simulink model "kuka_IMPC_lev2"  (R2022b)
settings: Solver=ode1  StartTime=0.0  StopTime=T_run  FixedStep=Ts  MaxStep=0.001  MinStep=0.0001  RelTol=1e-3
InitFcn:
  | kuka_IMPC_PriController_simulink_initial
StopFcn:
  | %Analyze%
values from neighbouring files (symbols this model uses):
  Xprime_r_lev1 = [Xprime_r_ini_stop_lev1 Xprime_r_lev1]    [Get_X_ref.m]
undefined symbols (not defined in the file or in its folder): A1_X_bar_lev1, A_QP, B1_dtau_bar_lev1, K_lev1, L1_tilde, L2_tilde, L_lev1, lb_QP, lbA_QP_ini, N, q_bar_sim_ini, q_ini, qd_ini, R_const_lev1, tau_sim_ini, Ts, ub_QP, ubA_QP_ini, x1_bar_sim_ini
libraries: robotmaniplib x8, cjt_library_models x1
settings Model: PauseTimes=7.5  Creator=ywang  LastModifiedBy=zheng
settings SolverCC: InitialStep=0.0001  AlgebraicLoopSolver=LineSearch
settings DataIOCC: ReturnWorkspaceOutputs=off
settings DebuggingCC: UnconnectedInputMsg=warning  UnconnectedOutputMsg=warning  UnconnectedLineMsg=warning  PregeneratedLibrarySubsystemCodeDiagnostic=none  SFMachineParentedDataDiag=warning  ArithmeticOperatorsInVariantConditions=warning
settings ModelReferenceCC: EnableRefExpFcnMdlSchedulingChecks=on
settings SFSimCC: SimUseLocalCustomCode=off  CustomCodeUndefinedFunction=UseInterfaceOnly
settings RTWCC: RTWUseLocalCustomCode=off  DLArmComputeVersion=19.05
settings CodeAppCC: StateflowObjectComments=on

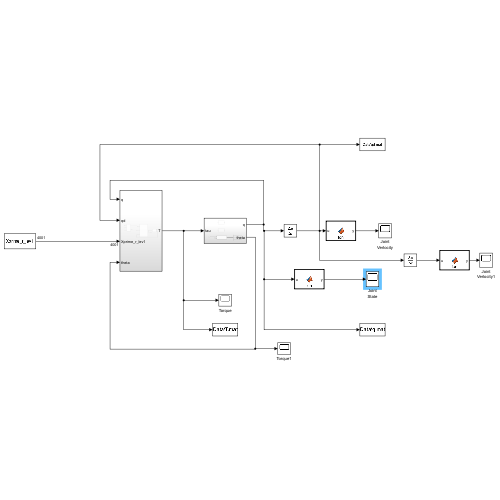
[thumbnail: Simulink's stored preview of the top-level diagram]
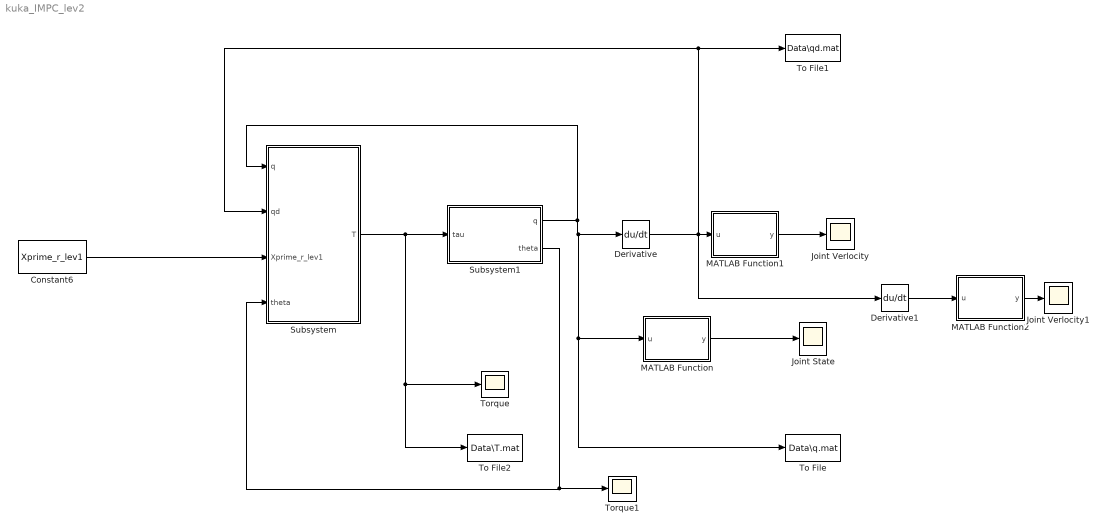
== system kuka_IMPC_lev2 ==
  Constant6 : Constant  Value=Xprime_r_lev1
  Derivative : Derivative
  Derivative1 : Derivative
  Joint State : Scope
  Joint Verlocity : Scope
  Joint Verlocity1 : Scope
  MATLAB Function : MATLAB Function  TreatAsAtomicUnit=on
  MATLAB Function1 : MATLAB Function  TreatAsAtomicUnit=on
  MATLAB Function2 : MATLAB Function  TreatAsAtomicUnit=on
  Subsystem : Subsystem
  Subsystem1 : Subsystem
  To File : ToFile  Filename=Data\q.mat  MatrixName=q
  To File1 : ToFile  Filename=Data\qd.mat  MatrixName=qd
  To File2 : ToFile  Filename=Data\T.mat  MatrixName=T
  Torque : Scope
  Torque1 : Scope
  wires:
  Subsystem/1(T) -> Torque/1, To File2/1, Subsystem1/1(tau)
  Constant6/1 -> Subsystem/3(Xprime_r_lev1)
  Subsystem1/1(q) -> Derivative/1, MATLAB Function/1(u), To File/1, Subsystem/1(q)
  MATLAB Function/1(y) -> Joint State/1
  MATLAB Function1/1(y) -> Joint Verlocity/1
  MATLAB Function2/1(y) -> Joint Verlocity1/1
  Derivative/1 -> Derivative1/1, MATLAB Function1/1(u), To File1/1, Subsystem/2(qd)
  Derivative1/1 -> MATLAB Function2/1(u)
  Subsystem1/2(theta) -> Torque1/1, Subsystem/4(theta)

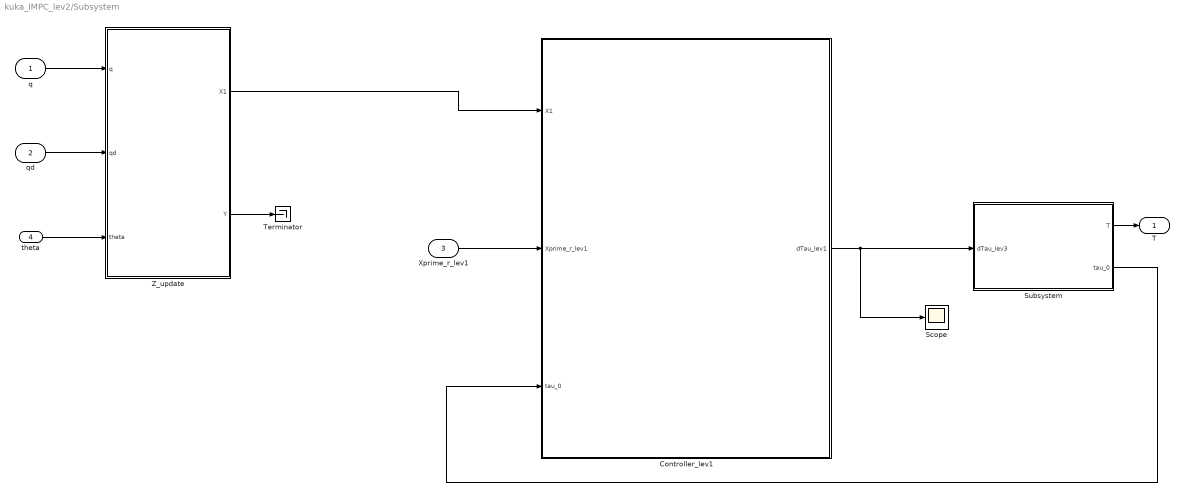
== system kuka_IMPC_lev2/Subsystem ==
  q : Inport
  qd : Inport  Port=2
  Xprime_r_lev1 : Inport  Port=3
  theta : Inport  Port=4
  Controller_lev1 : Subsystem
  Scope : Scope
  Subsystem : Subsystem
  Terminator : Terminator
  Z_update : Subsystem
  T : Outport
  wires:
  q/1 -> Z_update/1(q)
  qd/1 -> Z_update/2(qd)
  Z_update/1(X1) -> Controller_lev1/1(X1)
  Xprime_r_lev1/1 -> Controller_lev1/2(Xprime_r_lev1)
  Subsystem/1(T) -> T/1
  Subsystem/2(tau_0) -> Controller_lev1/3(tau_0)
  Z_update/2(Y) -> Terminator/1
  Controller_lev1/1(dTau_lev1) -> Subsystem/1(dTau_lev3), Scope/1
  theta/1 -> Z_update/3(theta)

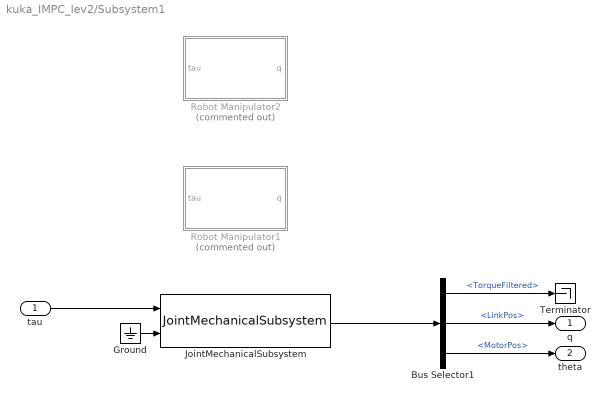
== system kuka_IMPC_lev2/Subsystem1 ==
  tau : Inport
  Bus Selector1 : BusSelector  OutputSignals=TorqueFiltered,LinkPos,MotorPos
  Ground : Ground
  JointMechanicalSubsystem : cjt_library_models/Joint models/JointMechanicalSubsystem  jointObj=exJoint  fc_vel=1000  fc_torque=1000  input_delay=0  output_delay=1  quantize=off  quantize_bits=19  input_noise_enabled=off  output_noise_enabled=off  var_u=0  var_y=1.8e-10
  Robot Manipulator1 : Subsystem  Commented=on
  Robot Manipulator2 : Subsystem  Commented=on
  Terminator : Terminator
  q : Outport
  theta : Outport  Port=2
  wires:
  Bus Selector1/1 -> Terminator/1  "<TorqueFiltered>"
  JointMechanicalSubsystem/1 -> Bus Selector1/1
  Ground/1 -> JointMechanicalSubsystem/2
  tau/1 -> JointMechanicalSubsystem/1
  Bus Selector1/2 -> q/1  "<LinkPos>"
  Bus Selector1/3 -> theta/1  "<MotorPos>"

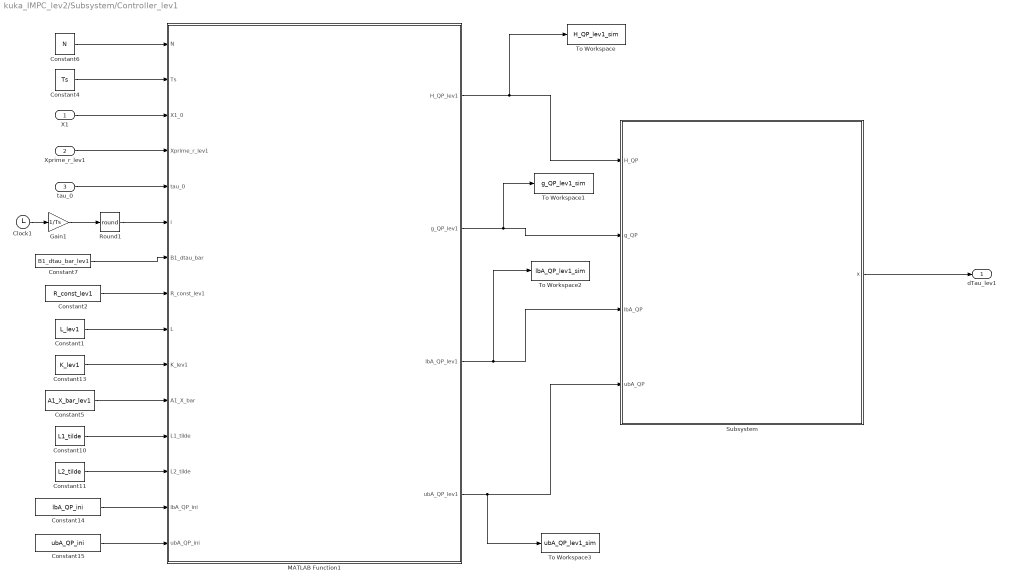
== system kuka_IMPC_lev2/Subsystem/Controller_lev1 ==
  X1 : Inport
  Xprime_r_lev1 : Inport  Port=2
  tau_0 : Inport  Port=3
  Clock1 : Clock
  Constant1 : Constant  Value=L_lev1
  Constant10 : Constant  Value=L1_tilde
  Constant11 : Constant  Value=L2_tilde
  Constant13 : Constant  Value=K_lev1
  Constant14 : Constant  Value=lbA_QP_ini
  Constant15 : Constant  Value=ubA_QP_ini
  Constant2 : Constant  Value=R_const_lev1
  Constant4 : Constant  Value=Ts
  Constant5 : Constant  Value=A1_X_bar_lev1
  Constant6 : Constant  Value=N
  Constant7 : Constant  Value=B1_dtau_bar_lev1
  Gain1 : Gain  Gain=1/Ts
  MATLAB Function1 : MATLAB Function  TreatAsAtomicUnit=on
  Round1 : Rounding  Operator=round
  Subsystem : Subsystem
  To Workspace : ToWorkspace  VariableName=H_QP_lev1_sim  SaveFormat=Timeseries  SampleTime=-1
  To Workspace1 : ToWorkspace  VariableName=g_QP_lev1_sim  SaveFormat=Timeseries  SampleTime=-1
  To Workspace2 : ToWorkspace  VariableName=lbA_QP_lev1_sim  SaveFormat=Timeseries  SampleTime=-1
  To Workspace3 : ToWorkspace  VariableName=ubA_QP_lev1_sim  SaveFormat=Timeseries  SampleTime=-1
  dTau_lev1 : Outport
  wires:
  Constant4/1 -> MATLAB Function1/2(Ts)
  Constant1/1 -> MATLAB Function1/9(L)
  Constant5/1 -> MATLAB Function1/11(A1_X_bar)
  Constant11/1 -> MATLAB Function1/13(L2_tilde)
  Constant10/1 -> MATLAB Function1/12(L1_tilde)
  MATLAB Function1/1(H_QP_lev1) -> To Workspace/1, Subsystem/1(H_QP)
  MATLAB Function1/2(g_QP_lev1) -> To Workspace1/1, Subsystem/2(g_QP)
  Clock1/1 -> Gain1/1
  Gain1/1 -> Round1/1
  Xprime_r_lev1/1 -> MATLAB Function1/4(Xprime_r_lev1)
  Constant13/1 -> MATLAB Function1/10(K_lev1)
  Constant14/1 -> MATLAB Function1/14(lbA_QP_ini)
  Constant15/1 -> MATLAB Function1/15(ubA_QP_ini)
  X1/1 -> MATLAB Function1/3(X1_0)
  tau_0/1 -> MATLAB Function1/5(tau_0)
  Constant6/1 -> MATLAB Function1/1(N)
  Subsystem/1(x) -> dTau_lev1/1
  MATLAB Function1/3(lbA_QP_lev1) -> To Workspace2/1, Subsystem/3(lbA_QP)
  MATLAB Function1/4(ubA_QP_lev1) -> To Workspace3/1, Subsystem/4(ubA_QP)
  Constant7/1 -> MATLAB Function1/7(B1_dtau_bar)
  Constant2/1 -> MATLAB Function1/8(R_const_lev1)
  Round1/1 -> MATLAB Function1/6(i)

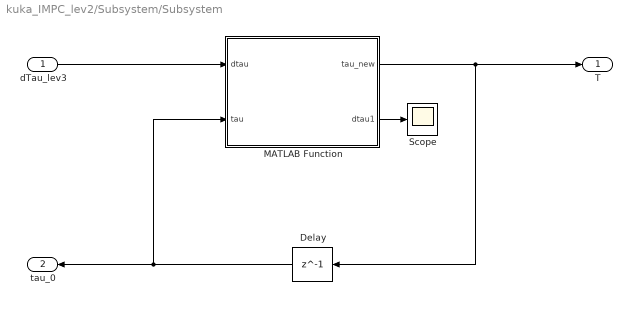
== system kuka_IMPC_lev2/Subsystem/Subsystem ==
  dTau_lev3 : Inport
  Delay : Delay  DelayLength=1  InitialCondition=tau_sim_ini
  MATLAB Function : MATLAB Function  TreatAsAtomicUnit=on
  Scope : Scope
  T : Outport
  tau_0 : Outport  Port=2
  wires:
  dTau_lev3/1 -> MATLAB Function/1(dtau)
  Delay/1 -> tau_0/1, MATLAB Function/2(tau)
  MATLAB Function/1(tau_new) -> Delay/1, T/1
  MATLAB Function/2(dtau1) -> Scope/1

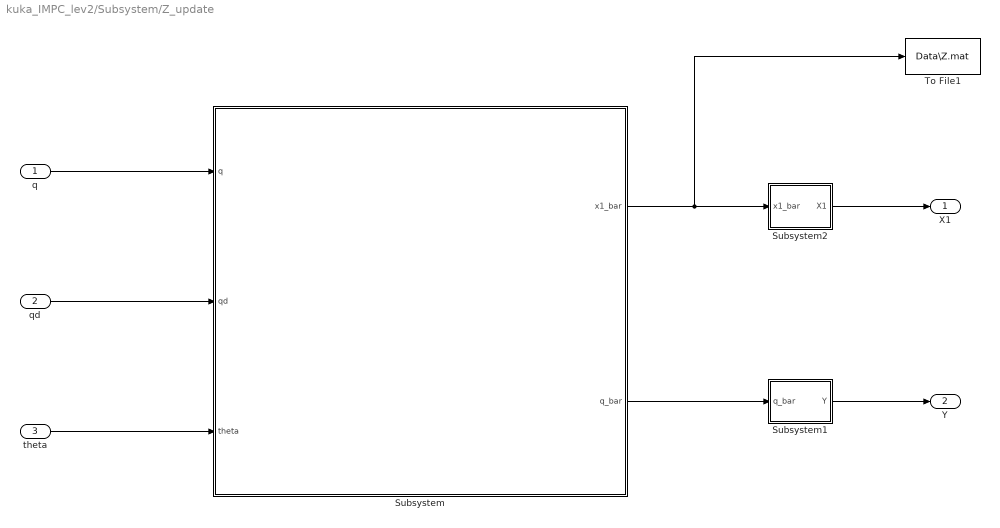
== system kuka_IMPC_lev2/Subsystem/Z_update ==
  q : Inport
  qd : Inport  Port=2
  theta : Inport  Port=3
  Subsystem : Subsystem
  Subsystem1 : Subsystem
  Subsystem2 : Subsystem
  To File1 : ToFile  Filename=Data\Z.mat  MatrixName=Z
  X1 : Outport
  Y : Outport  Port=2
  wires:
  qd/1 -> Subsystem/2(qd)
  q/1 -> Subsystem/1(q)
  Subsystem1/1(Y) -> Y/1
  Subsystem/2(q_bar) -> Subsystem1/1(q_bar)
  Subsystem2/1(X1) -> X1/1
  Subsystem/1(x1_bar) -> To File1/1, Subsystem2/1(x1_bar)
  theta/1 -> Subsystem/3(theta)

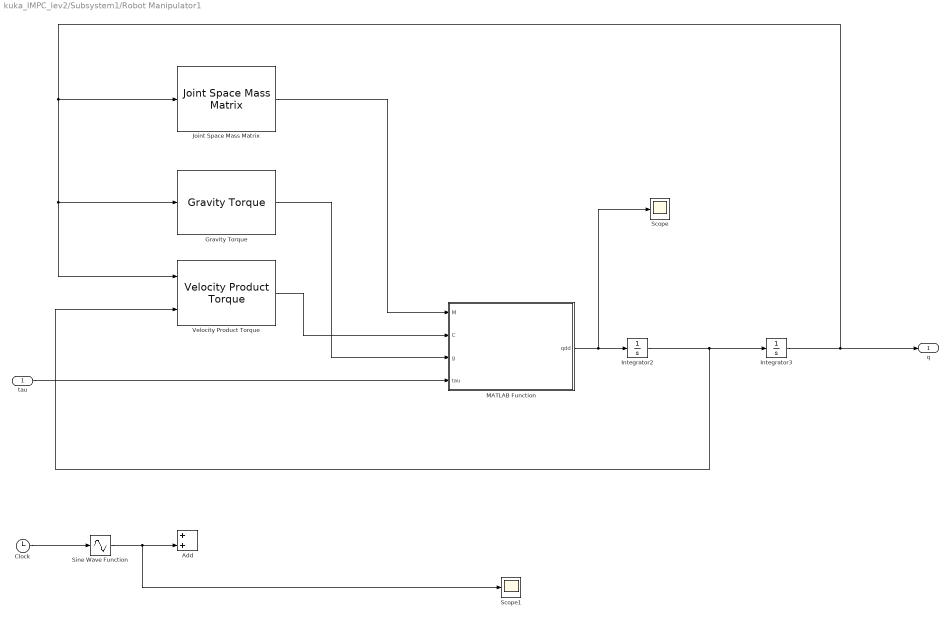
== system kuka_IMPC_lev2/Subsystem1/Robot Manipulator1 ==
  tau : Inport
  Add : Sum
  Clock : Clock
  Gravity Torque : robotmaniplib/Gravity Torque  RigidBodyTree=kuka  SimulateUsing=Interpreted execution
  Integrator2 : Integrator  InitialCondition=qd_ini  ContinuousStateAttributes='velocity'
  Integrator3 : Integrator  InitialCondition=q_ini  ContinuousStateAttributes='position'
  Joint Space Mass Matrix : robotmaniplib/Joint Space Mass Matrix  RigidBodyTree=kuka  SimulateUsing=Interpreted execution
  MATLAB Function : MATLAB Function  TreatAsAtomicUnit=on
  Scope : Scope
  Scope1 : Scope
  Sine Wave Function : Sin  TimeSource=Use external signal  Amplitude=0.5  Frequency=2  SampleTime=0
  Velocity Product Torque : robotmaniplib/Velocity Product Torque  RigidBodyTree=kuka  SimulateUsing=Interpreted execution
  q : Outport  VectorParamsAs1DForOutWhenUnconnected=off
  wires:
  Integrator3/1 -> q/1, Velocity Product Torque/1, Gravity Torque/1, Joint Space Mass Matrix/1
  Integrator2/1 -> Integrator3/1, Velocity Product Torque/2
  Joint Space Mass Matrix/1 -> MATLAB Function/1(M)
  MATLAB Function/1(qdd) -> Scope/1, Integrator2/1
  Velocity Product Torque/1 -> MATLAB Function/2(C)
  Gravity Torque/1 -> MATLAB Function/3(g)
  Sine Wave Function/1 -> Scope1/1, Add/2
  Clock/1 -> Sine Wave Function/1
  tau/1 -> MATLAB Function/4(tau)

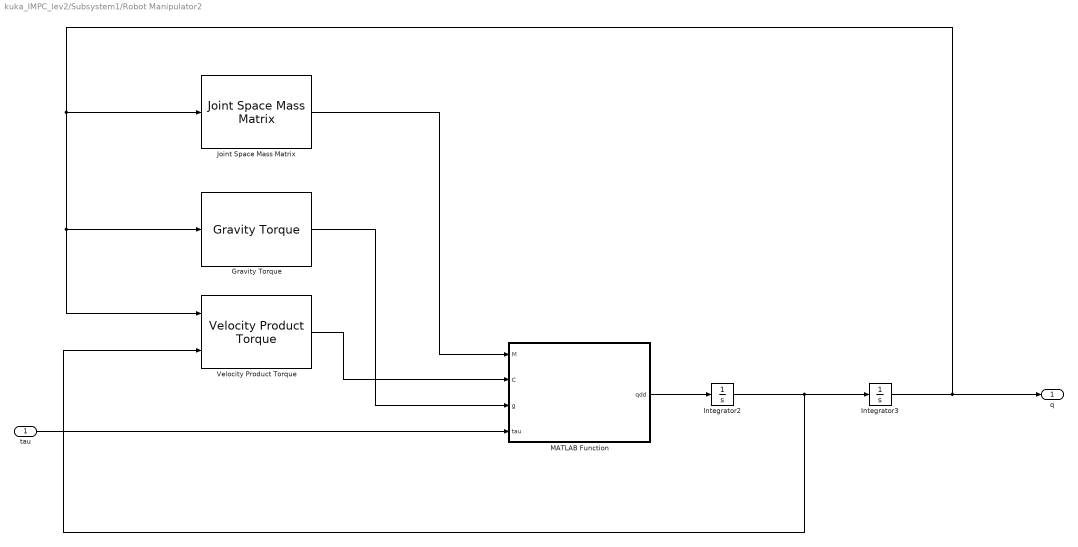
== system kuka_IMPC_lev2/Subsystem1/Robot Manipulator2 ==
  tau : Inport
  Gravity Torque : robotmaniplib/Gravity Torque  RigidBodyTree=kuka  SimulateUsing=Interpreted execution
  Integrator2 : Integrator  InitialCondition=qd_ini  ContinuousStateAttributes='velocity'
  Integrator3 : Integrator  InitialCondition=q_ini  ContinuousStateAttributes='position'
  Joint Space Mass Matrix : robotmaniplib/Joint Space Mass Matrix  RigidBodyTree=kuka  SimulateUsing=Interpreted execution
  MATLAB Function : MATLAB Function  TreatAsAtomicUnit=on
  Velocity Product Torque : robotmaniplib/Velocity Product Torque  RigidBodyTree=kuka  SimulateUsing=Interpreted execution
  q : Outport  VectorParamsAs1DForOutWhenUnconnected=off
  wires:
  Integrator3/1 -> q/1, Velocity Product Torque/1, Gravity Torque/1, Joint Space Mass Matrix/1
  Integrator2/1 -> Integrator3/1, Velocity Product Torque/2
  Joint Space Mass Matrix/1 -> MATLAB Function/1(M)
  MATLAB Function/1(qdd) -> Integrator2/1
  Velocity Product Torque/1 -> MATLAB Function/2(C)
  Gravity Torque/1 -> MATLAB Function/3(g)
  tau/1 -> MATLAB Function/4(tau)

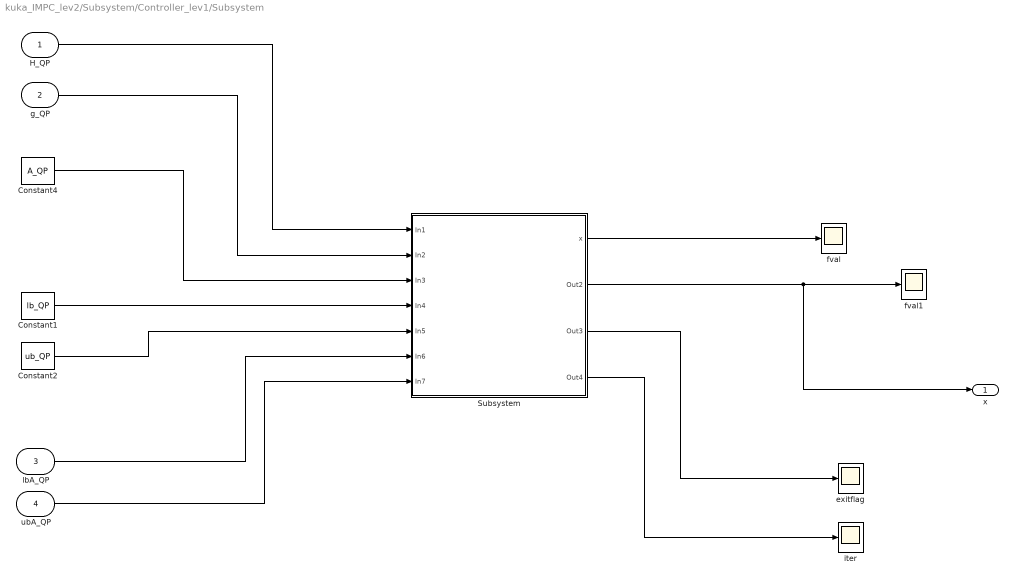
== system kuka_IMPC_lev2/Subsystem/Controller_lev1/Subsystem ==
  H_QP : Inport  PortDimensions=9
  g_QP : Inport  Port=2  PortDimensions=3
  lbA_QP : Inport  Port=3  PortDimensions=9
  ubA_QP : Inport  Port=4  PortDimensions=9
  Constant1 : Constant  Value=lb_QP
  Constant2 : Constant  Value=ub_QP
  Constant4 : Constant  Value=A_QP
  Subsystem : Subsystem
  exitflag : Scope
  fval : Scope
  fval1 : Scope
  iter : Scope
  x : Outport
  wires:
  Subsystem/2(Out2) -> x/1, fval1/1
  H_QP/1 -> Subsystem/1(In1)
  g_QP/1 -> Subsystem/2(In2)
  Constant4/1 -> Subsystem/3(In3)
  lbA_QP/1 -> Subsystem/6(In6)
  ubA_QP/1 -> Subsystem/7(In7)
  Subsystem/1(x) -> fval/1
  Subsystem/3(Out3) -> exitflag/1
  Subsystem/4(Out4) -> iter/1
  Constant1/1 -> Subsystem/4(In4)
  Constant2/1 -> Subsystem/5(In5)

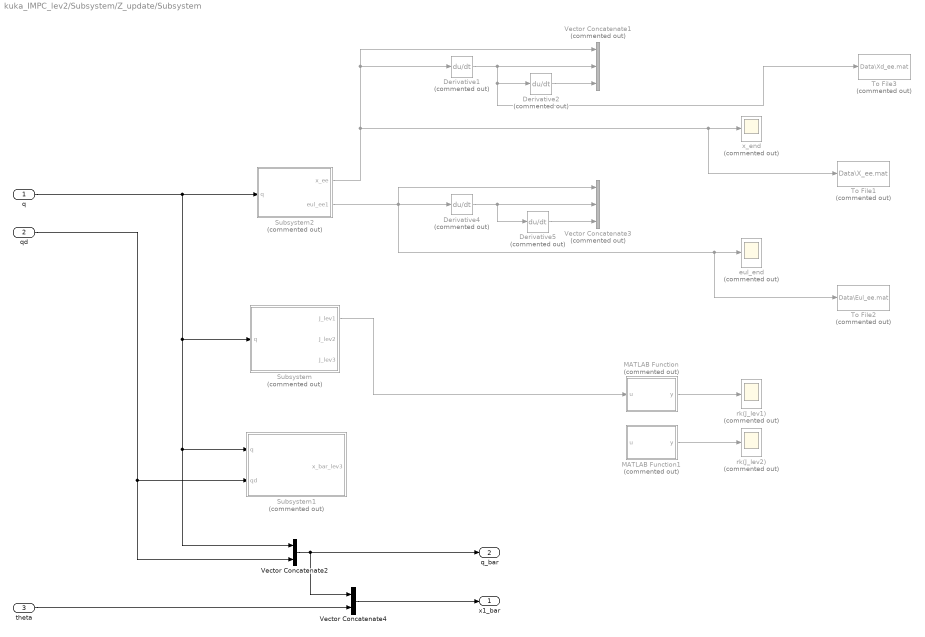
== system kuka_IMPC_lev2/Subsystem/Z_update/Subsystem ==
  q : Inport
  qd : Inport  Port=2
  theta : Inport  Port=3
  Derivative{1..2,4..5} (4 alike) : Derivative  Commented=on
  MATLAB Function : MATLAB Function  Commented=on  TreatAsAtomicUnit=on
  MATLAB Function1 : MATLAB Function  Commented=on  TreatAsAtomicUnit=on
  Subsystem : Subsystem  Commented=on
  Subsystem1 : Subsystem  Commented=on
  Subsystem2 : Subsystem  Commented=on
  To File1 : ToFile  Commented=on  Filename=Data\X_ee.mat  MatrixName=x_ee
  To File2 : ToFile  Commented=on  Filename=Data\Eul_ee.mat  MatrixName=eul_ee
  To File3 : ToFile  Commented=on  Filename=Data\Xd_ee.mat  MatrixName=xd_ee
  Vector Concatenate1 : Concatenate  Commented=on  NumInputs=3
  Vector Concatenate2 : Concatenate
  Vector Concatenate3 : Concatenate  Commented=on  NumInputs=3
  Vector Concatenate4 : Concatenate
  eul_end : Scope  Commented=on
  rk(J_lev1) : Scope  Commented=on
  rk(J_lev2) : Scope  Commented=on
  x_end : Scope  Commented=on
  x1_bar : Outport
  q_bar : Outport  Port=2
  wires:
  q/1 -> Subsystem2/1(q), Subsystem/1(q), Subsystem1/1(q), Vector Concatenate2/1
  Vector Concatenate2/1 -> Vector Concatenate4/1, q_bar/1
  qd/1 -> Vector Concatenate2/2, Subsystem1/2(qd)
  Derivative1/1 -> To File3/1, Derivative2/1, Vector Concatenate1/2
  Derivative2/1 -> Vector Concatenate1/3
  Subsystem/1(J_lev1) -> MATLAB Function/1(u)
  Subsystem2/1(x_ee) -> Derivative1/1, Vector Concatenate1/1, To File1/1, x_end/1
  Derivative5/1 -> Vector Concatenate3/3
  Derivative4/1 -> Derivative5/1, Vector Concatenate3/2
  Subsystem2/2(eul_ee1) -> To File2/1, eul_end/1, Derivative4/1, Vector Concatenate3/1
  MATLAB Function/1(y) -> rk(J_lev1)/1
  MATLAB Function1/1(y) -> rk(J_lev2)/1
  theta/1 -> Vector Concatenate4/2
  Vector Concatenate4/1 -> x1_bar/1

== system kuka_IMPC_lev2/Subsystem/Z_update/Subsystem1 ==
  q_bar : Inport
  Delay1 : Delay  DelayLength=1  InitialCondition=q_bar_sim_ini
  Vector Concatenate2 : Concatenate
  Y : Outport
  wires:
  Delay1/1 -> Vector Concatenate2/2
  q_bar/1 -> Delay1/1, Vector Concatenate2/1
  Vector Concatenate2/1 -> Y/1

== system kuka_IMPC_lev2/Subsystem/Z_update/Subsystem2 ==
  x1_bar : Inport
  Delay : Delay  DelayLength=1  InitialCondition=x1_bar_sim_ini
  Vector Concatenate1 : Concatenate
  X1 : Outport
  wires:
  Delay/1 -> Vector Concatenate1/2
  x1_bar/1 -> Delay/1, Vector Concatenate1/1
  Vector Concatenate1/1 -> X1/1

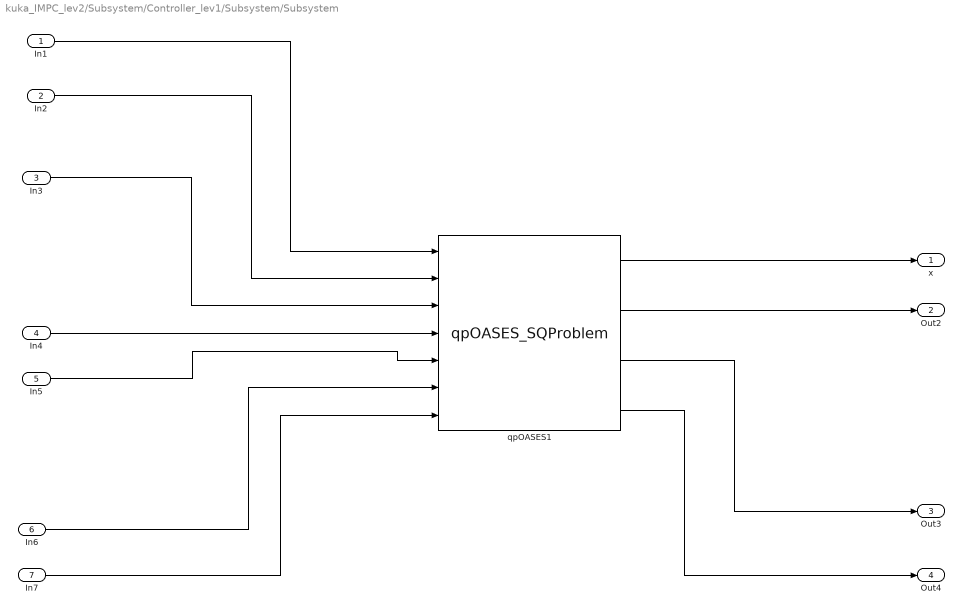
== system kuka_IMPC_lev2/Subsystem/Controller_lev1/Subsystem/Subsystem ==
  In1 : Inport
  In2 : Inport  Port=2
  In3 : Inport  Port=3
  In4 : Inport  Port=4
  In5 : Inport  Port=5
  In6 : Inport  Port=6
  In7 : Inport  Port=7
  qpOASES1 : S-Function  FunctionName=qpOASES_SQProblem  SFunctionDeploymentMode=off  EnableBusSupport=off
  x : Outport
  Out2 : Outport  Port=2
  Out3 : Outport  Port=3
  Out4 : Outport  Port=4
  wires:
  qpOASES1/4 -> Out4/1
  In1/1 -> qpOASES1/1
  qpOASES1/3 -> Out3/1
  In2/1 -> qpOASES1/2
  In7/1 -> qpOASES1/7
  In4/1 -> qpOASES1/4
  In3/1 -> qpOASES1/3
  qpOASES1/2 -> Out2/1
  qpOASES1/1 -> x/1
  In6/1 -> qpOASES1/6
  In5/1 -> qpOASES1/5

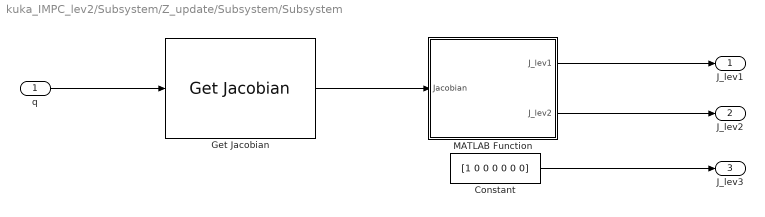
== system kuka_IMPC_lev2/Subsystem/Z_update/Subsystem/Subsystem ==
  q : Inport
  Constant : Constant  Value=[1 0 0 0 0 0 0]
  Get Jacobian : robotmaniplib/Get Jacobian  RigidBodyTree=kuka  EndEffector=iiwa_link_ee_kuka  SimulateUsing=Interpreted execution
  MATLAB Function : MATLAB Function  TreatAsAtomicUnit=on
  J_lev1 : Outport
  J_lev2 : Outport  Port=2
  J_lev3 : Outport  Port=3
  wires:
  q/1 -> Get Jacobian/1
  Get Jacobian/1 -> MATLAB Function/1(Jacobian)
  MATLAB Function/1(J_lev1) -> J_lev1/1
  MATLAB Function/2(J_lev2) -> J_lev2/1
  Constant/1 -> J_lev3/1

== system kuka_IMPC_lev2/Subsystem/Z_update/Subsystem/Subsystem1 ==
  q : Inport
  qd : Inport  Port=2
  Derivative6 : Derivative
  MATLAB Function : MATLAB Function  TreatAsAtomicUnit=on
  x_bar_lev3 : Outport
  wires:
  MATLAB Function/1(x_lev3) -> x_bar_lev3/1
  q/1 -> MATLAB Function/1(q)
  qd/1 -> Derivative6/1, MATLAB Function/2(qd)
  Derivative6/1 -> MATLAB Function/3(qdd)

== system kuka_IMPC_lev2/Subsystem/Z_update/Subsystem/Subsystem2 ==
  q : Inport
  Get Transform : robotmaniplib/Get Transform  RigidBodyTree=kuka  SourceBody=iiwa_link_ee_kuka  TargetBody=world  SimulateUsing=Interpreted execution
  MATLAB Function : MATLAB Function  TreatAsAtomicUnit=on
  MATLAB Function1 : MATLAB Function  TreatAsAtomicUnit=on
  x_ee : Outport
  eul_ee1 : Outport  Port=2
  wires:
  q/1 -> Get Transform/1
  Get Transform/1 -> MATLAB Function1/1(T), MATLAB Function/1(T)
  MATLAB Function/1(x_ee) -> x_ee/1
  MATLAB Function1/1(eul_ee) -> eul_ee1/1

== matlab function kuka_IMPC_lev2/MATLAB Function1 ==
  data: u input; y output
function y = fcn(u)

y = (180/pi) * u;

== matlab function kuka_IMPC_lev2/Subsystem/Z_update/Subsystem/Subsystem1/MATLAB Function ==
  data: q input; x_lev3 output; qd input; qdd input
function x_lev3 = f(q,qd,qdd)
    x_lev3 = [  q(1);
               qd(1);
              qdd(1)];
          

end

== matlab function kuka_IMPC_lev2/Subsystem/Controller_lev1/MATLAB Function1 ==
  data: N input; Ts input; H_QP_lev1 output; X1_0 input; Xprime_r_lev1 input; tau_0 input; i input; B1_dtau_bar input; R_const_lev1 input; L input; K_lev1 input; A1_X_bar input; L1_tilde input; L2_tilde input; g_QP_lev1 output; lbA_QP_lev1 output; ubA_QP_lev1 output; lbA_QP_ini input; ubA_QP_ini input
function [H_QP_lev1, g_QP_lev1, lbA_QP_lev1, ubA_QP_lev1] = QP_parameter_lev1(N,Ts, X1_0, Xprime_r_lev1,tau_0,i,B1_dtau_bar,R_const_lev1,L,K_lev1,A1_X_bar,L1_tilde,L2_tilde,lbA_QP_ini,ubA_QP_ini)
    k = 3;

    tau_0_bar = repmat(tau_0,k,1); 
    Xr_prime = Xprime_r_lev1(i+1:i+k);
    v = reshape(Xr_prime,N,1);
    G = K_lev1*v;
%     Fe = repmat(Fe,k,1);
%     
%     B1_dtau = Get_B1_dtau(Ts,M_bar_inv, J_lev1);  
%     B1_dtau_bar = Formulate_N_RecurMat(N, A1_X,B1_dtau);
%     
%     H = 2*R_const*eye(7*k)+2*B1_dtau_bar'*L*B1_dtau_bar;
%     H_QP_lev1 = reshape(H,7*k*7*k,1); 
    
    H = 2*R_const_lev1*eye(k)+2*B1_dtau_bar'*L*B1_dtau_bar;
    H_QP_lev1 = reshape(H,k*k,1);

%     g_QP_lev1 = 2*eye(k)*B1_dtau_bar'*(L'*A1_X_bar*X1_0-G);
    g_QP_lev1_temp = 2*eye(k)*B1_dtau_bar'*(L'*A1_X_bar*X1_0-G);
    g_QP_lev1 = reshape(g_QP_lev1_temp,k,1);

    % with qd constraints
    lbA_QP_lev1_temp = lbA_QP_ini-[L1_tilde*X1_0;
                              L2_tilde*X1_0;
                                 tau_0_bar];
    lbA_QP_lev1 = reshape(lbA_QP_lev1_temp,3*k,1);
    ubA_QP_lev1_temp = ubA_QP_ini-[L1_tilde*X1_0;
                              L2_tilde*X1_0;
                                 tau_0_bar];
    ubA_QP_lev1 = reshape(ubA_QP_lev1_temp,3*k,1);
                        
%     % without qd constraints
%     lbA_QP = lbA_QP_ini-[L1_tilde*Y_0;
%                             tau_0_bar];
%     ubA_QP = ubA_QP_ini-[L1_tilde*Y_0;
%                             tau_0_bar];
%                    
%                             
%   
    
end

== matlab function kuka_IMPC_lev2/Subsystem/Z_update/Subsystem/MATLAB Function ==
  data: u input; y output
function y = fcn(u)

y = rank(u);

== matlab function kuka_IMPC_lev2/Subsystem/Z_update/Subsystem/MATLAB Function1 ==
  data: u input; y output
function y = fcn(u)

y = rank(u);

== matlab function kuka_IMPC_lev2/MATLAB Function2 ==
  data: u input; y output
function y = fcn(u)

y = (180/pi) * u;

== matlab function kuka_IMPC_lev2/Subsystem1/Robot Manipulator2/MATLAB Function ==
  data: M input; qdd output; C input; g input; tau input
function qdd = fcn(M,C,g,tau)
    qdd = M\(tau-C-g);
    
end

== matlab function kuka_IMPC_lev2/Subsystem/Z_update/Subsystem/Subsystem/MATLAB Function ==
  data: Jacobian input; J_lev1 output; J_lev2 output
function [J_lev1,J_lev2] = Get_J_lev(Jacobian)
    J_lev1 = Jacobian(4:6,:);
    J_lev2 = Jacobian(1:3,:);

    
end

== matlab function kuka_IMPC_lev2/Subsystem/Z_update/Subsystem/Subsystem2/MATLAB Function ==
  data: T input; x_ee output
function x_ee = T2x_ee(T)
x_ee = T(1:3,4);

== matlab function kuka_IMPC_lev2/Subsystem1/Robot Manipulator1/MATLAB Function ==
  data: M input; qdd output; C input; g input; tau input
function qdd = fcn(M,C,g,tau)
    M = M+M*0.5;
    qdd = M\(tau-C-g);
    
end

== matlab function kuka_IMPC_lev2/MATLAB Function ==
  data: u input; y output
function y = fcn(u)

y = (180/pi) * u;

== matlab function kuka_IMPC_lev2/Subsystem/Subsystem/MATLAB Function ==
  data: dtau input; tau_new output; tau input; dtau1 output
function [tau_new,dtau1] = fcn(dtau,tau)
tau_new = tau+dtau(1);
dtau1 = dtau(1);
end

== matlab function kuka_IMPC_lev2/Subsystem/Z_update/Subsystem/Subsystem2/MATLAB Function1 ==
  data: T input; eul_ee output
function eul_ee = T2eul_ee(T)
    eul_ee = rotm2eul(T(1:3,1:3),'XYZ')';

end
